simulink model "airspeed_from_pitch_loop_correct"  (Simulink 8.2)
settings: Solver=ode45  StartTime=0.0  StopTime=100  RelTol=1e-3
values from neighbouring files (symbols this model uses):
  a_theta1 = den(2)    [computeGains.m]
  a_theta2 = den(3)    [computeGains.m]
  a_theta3 = num(3)    [computeGains.m]
  a_V1 = den(2)    [computeGains.m]
  delta_e_max = 45*pi/180    (= 0.785398163397)    [computeGains.m]
undefined symbols (not defined in the file or in its folder): P
settings Model: Creator=beard  LastModifiedBy=ecestudent

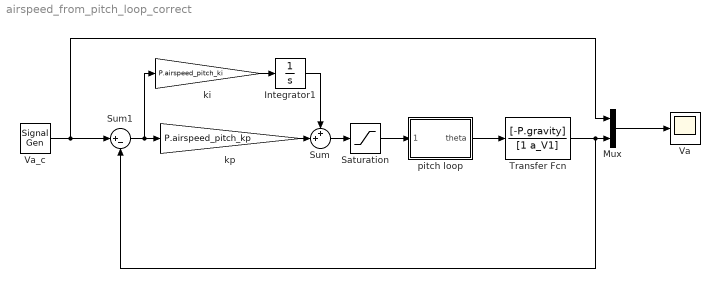
== system airspeed_from_pitch_loop_correct ==
  Integrator1 : Integrator
  Mux : Mux  Inputs=2
  Saturation : Saturate  UpperLimit=30*pi/180/P.K_theta_DC  LowerLimit=-30*pi/180/P.K_theta_DC
  Sum : Sum  Inputs=++|
  Sum1 : Sum  Inputs=|+-
  Transfer Fcn : TransferFcn  Numerator=[-P.gravity]  Denominator=[1 a_V1]
  Va : Scope
      settings: TimeRange=100  YMin=-10  YMax=15
  Va_c : SignalGenerator  WaveForm=square  Amplitude=5  Frequency=.02
  ki : Gain  Gain=P.airspeed_pitch_ki
  kp : Gain  Gain=P.airspeed_pitch_kp
  pitch loop : Subsystem
  wires:
  Sum/1 -> Saturation/1
  kp/1 -> Sum/2
  ki/1 -> Integrator1/1
  Integrator1/1 -> Sum/1
  Va_c/1 -> Sum1/1, Mux/1
  Mux/1 -> Va/1
  pitch loop/1(theta) -> Transfer Fcn/1
  Transfer Fcn/1 -> Mux/2, Sum1/2
  Saturation/1 -> pitch loop/1(theta_c)
  Sum1/1 -> ki/1, kp/1

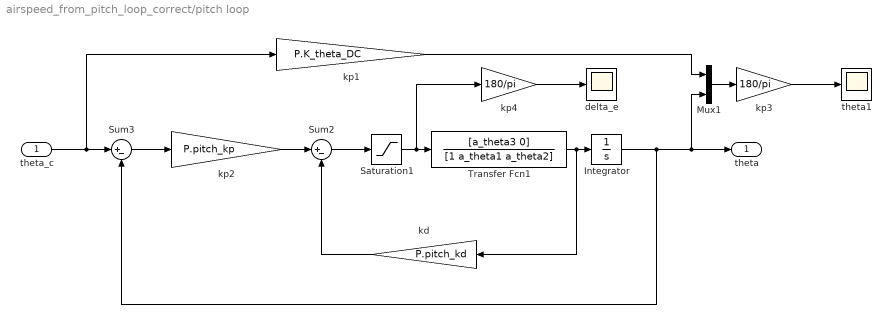
== system airspeed_from_pitch_loop_correct/pitch loop ==
  theta_c : Inport
  Integrator : Integrator
  Mux1 : Mux  Inputs=2
  Saturation1 : Saturate  UpperLimit=delta_e_max  LowerLimit=-delta_e_max
  Sum2 : Sum  Inputs=|+-
  Sum3 : Sum  Inputs=|+-
  Transfer Fcn1 : TransferFcn  Numerator=[a_theta3 0]  Denominator=[1 a_theta1 a_theta2]
  delta_e : Scope
      settings: TimeRange=100  YMin=-10  YMax=15
  kd : Gain  Gain=P.pitch_kd
  kp1 : Gain  Gain=P.K_theta_DC
  kp2 : Gain  Gain=P.pitch_kp
  kp3 : Gain  Gain=180/pi
  kp4 : Gain  Gain=180/pi
  theta1 : Scope
      settings: TimeRange=100  YMin=-40  YMax=40  SaveName=ScopeData2
  theta : Outport
  wires:
  Transfer Fcn1/1 -> Integrator/1, kd/1
  Saturation1/1 -> Transfer Fcn1/1, kp4/1
  Sum2/1 -> Saturation1/1
  Sum3/1 -> kp2/1
  Integrator/1 -> Sum3/2, Mux1/2, theta/1
  theta_c/1 -> Sum3/1, kp1/1
  Mux1/1 -> kp3/1
  kp4/1 -> delta_e/1
  kp2/1 -> Sum2/1
  kd/1 -> Sum2/2
  kp3/1 -> theta1/1
  kp1/1 -> Mux1/1
